simulink model "ECM_second_plot"  (R2019b)
settings: Solver=ode4  StartTime=0.0  StopTime=max(Time_new)  FixedStep=0.05  RelTol=1e-3
values from neighbouring files (symbols this model uses):
  c1_calib = xopt(1)    [RCID_Single_Temp_Model_v3_mod.m]
  c2_calib = xopt(3)    [RCID_Single_Temp_Model_v3_mod.m]
  I_new = -1*I(Pulse_Start_Index(SOC_test)-5:Pulse_Start_Index(SOC_test)+Smallest_Pulse-1)    [RCID_Single_Temp_Model_old.m]    (also in RCID_Single_Temp_Model_v2.m; RCID_Single_Temp_Model_v3_mod.m = TestData.I(Pulse_Start_Index(i) : Pulse_Stop_Index(i)+300))
  ini_SOC_opt = SOC_count(Pulse_Start_Index(i))    [RCID_Single_Temp_Model_v3_mod.m]
  OCV = V(Initial_Pulse_Index)    [RCID_Single_Temp_Model_v3_mod.m]
  R0 = (abs((V_new(1) - V_new(2)) ./ (I_new(1) - I_new(end))))    [RCID_Single_Temp_Model_v3_mod.m]
  r1_calib = xopt(2)    [RCID_Single_Temp_Model_v3_mod.m]
  r2_calib = xopt(4)    [RCID_Single_Temp_Model_v3_mod.m]
  SOC = SOC_count(Initial_Pulse_Index)    [RCID_Single_Temp_Model_v3_mod.m]
  Time_new = Time(Pulse_Start_Index(SOC_test)-5:Pulse_Start_Index(SOC_test)+Smallest_Pulse-1)    [RCID_Single_Temp_Model_old.m]    (also in RCID_Single_Temp_Model_v2.m; RCID_Single_Temp_Model_v3_mod.m = TestData.Time(Pulse_Start_Index(i) : Pulse_Stop_Index(i)+300)
  V_new = V(Pulse_Start_Index(SOC_test)-5:Pulse_Start_Index(SOC_test)+Smallest_Pulse-1)    [RCID_Single_Temp_Model_old.m]    (also in RCID_Single_Temp_Model_v2.m; RCID_Single_Temp_Model_v3_mod.m = TestData.V(Pulse_Start_Index(i) : Pulse_Stop_Index(i)+300))
settings Model: Creator=yatin  LastModifiedBy=yatin

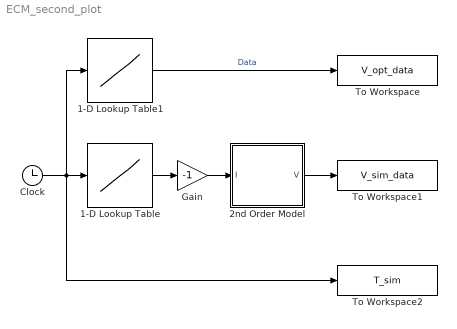
== system ECM_second_plot ==
  1-D Lookup Table : Lookup_n-D  NumberOfTableDimensions=1  BreakpointsForDimension1=Time_new  Table=I_new  InternalRulePriority=Speed  RndMeth=Simplest  InputSameDT=on
  1-D Lookup Table1 : Lookup_n-D  NumberOfTableDimensions=1  BreakpointsForDimension1=Time_new  Table=V_new  InternalRulePriority=Speed  RndMeth=Simplest  InputSameDT=on
  2nd Order Model : Subsystem
  Clock : Clock
  Gain : Gain  Gain=-1
  To Workspace : ToWorkspace  VariableName=V_opt_data  SampleTime=-1
  To Workspace1 : ToWorkspace  VariableName=V_sim_data  SampleTime=-1
  To Workspace2 : ToWorkspace  VariableName=T_sim  SampleTime=-1
  wires:
  Clock/1 -> 1-D Lookup Table1/1, To Workspace2/1, 1-D Lookup Table/1
  2nd Order Model/1(V) -> To Workspace1/1
  1-D Lookup Table1/1 -> To Workspace/1  "Data"
  1-D Lookup Table/1 -> Gain/1
  Gain/1 -> 2nd Order Model/1(I)

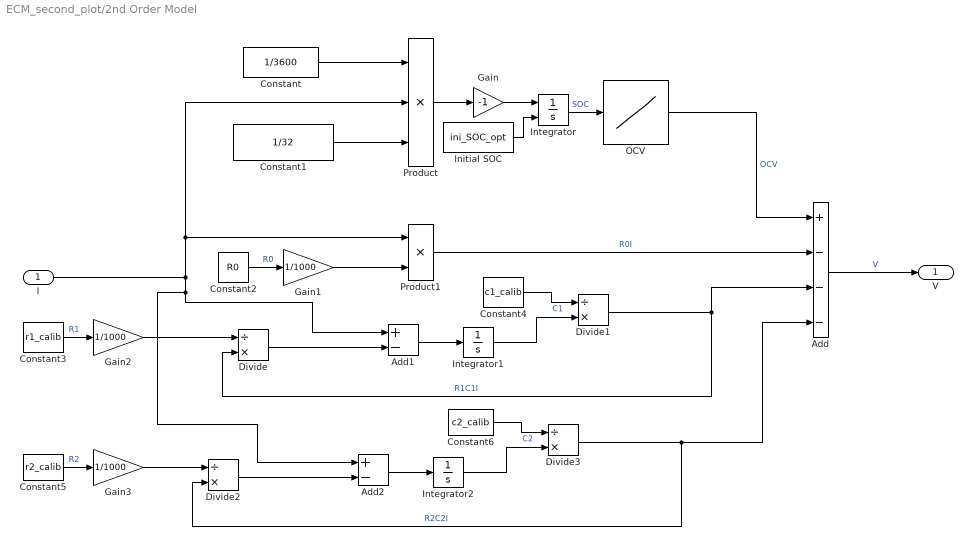
== system ECM_second_plot/2nd Order Model ==
  I : Inport
  Add : Sum  Inputs=+---
  Add1 : Sum  Inputs=+-
  Add2 : Sum  Inputs=+-
  Constant : Constant  Value=1/3600
  Constant1 : Constant  Value=1/32
  Constant2 : Constant  Value=R0
  Constant3 : Constant  Value=r1_calib
  Constant4 : Constant  Value=c1_calib
  Constant5 : Constant  Value=r2_calib
  Constant6 : Constant  Value=c2_calib
  Divide{,1..3} (4 alike) : Product  Inputs=/*
  Gain : Gain  Gain=-1
  Gain1 : Gain  Gain=1/1000
  Gain2 : Gain  Gain=1/1000
  Gain3 : Gain  Gain=1/1000
  Initial SOC : Constant  Value=ini_SOC_opt
  Integrator : Integrator  InitialConditionSource=external
  Integrator1 : Integrator  UpperSaturationLimit=1  LowerSaturationLimit=0
  Integrator2 : Integrator  UpperSaturationLimit=1  LowerSaturationLimit=0
  OCV : Lookup_n-D  NumberOfTableDimensions=1  BreakpointsForDimension1=flip(SOC)  Table=flip(OCV)  InternalRulePriority=Speed  RndMeth=Simplest  InputSameDT=on
  Product : Product  Inputs=3
  Product1 : Product
  V : Outport
  wires:
  Initial SOC/1 -> Integrator/2
  Constant1/1 -> Product/3
  Product/1 -> Gain/1
  Integrator/1 -> OCV/1  "SOC"
  OCV/1 -> Add/1  "OCV"
  Add/1 -> V/1  "V"
  Product1/1 -> Add/2  "R0I"
  Constant/1 -> Product/1
  Constant2/1 -> Gain1/1  "R0"
  Constant3/1 -> Gain2/1  "R1"
  Divide/1 -> Add1/2
  Add1/1 -> Integrator1/1
  Integrator1/1 -> Divide1/2
  Constant4/1 -> Divide1/1  "C1"
  Divide1/1 -> Divide/2, Add/3  "R1C1I"
  Divide3/1 -> Add/4, Divide2/2  "R2C2I"
  Constant6/1 -> Divide3/1  "C2"
  I/1 -> Add2/1, Add1/1, Product/2, Product1/1
  Add2/1 -> Integrator2/1
  Integrator2/1 -> Divide3/2
  Divide2/1 -> Add2/2
  Constant5/1 -> Gain3/1  "R2"
  Gain/1 -> Integrator/1
  Gain1/1 -> Product1/2
  Gain2/1 -> Divide/1
  Gain3/1 -> Divide2/1
